simulink model "Mmc"  (R2024b)
settings: Solver=ode23t  StartTime=0.0  StopTime=2  FixedStep=Ts_Power
values from neighbouring files (symbols this model uses):
  Ch = 0.94e-6*ones(4,3)    [MmcParameters.m]
  Cm = 0.55e-3    (= 0.00055)    [MmcParameters.m]
  Cmo = 0.55e-3*ones(4,3)    [MmcParameters.m]
  eta = N*delta_wmax*Vmax^2/(P_rated*sin(phi_r)-Q_rated*cos(phi_r))    [MmcParameters.m]
  Fnom = 50    [MmcParameters.m]
  fs = 20000    [MmcParameters.m]
  I_b = Snom/Vnom_AC/sqrt(3)    [MmcParameters.m]
  Ipp_b = Snom/Vnom_AC/sqrt(3/2)    [MmcParameters.m]
  kicir = R0*alpha_ic    (= 62831.8530718)    [MmcParameters.m]
  kpcir = L0*alpha_ic    (= 1012.64003201)    [MmcParameters.m]
  L0 = (4.67e-3+5e-3)    (= 0.00967)    [MmcParameters.m]
  mu = eta*4/((2*Vmax^2-V0^2)^2-V0^4)*(P_rated*cos(phi_r)+Q_rated*sin(phi_r))/N    [MmcParameters.m]
  Nb_PM = 2    [MmcParameters.m]
  phi_r = pi/2    (= 1.57079632679)    [MmcParameters.m]
  R0 = 0.1+0.5    (= 0.6)    [MmcParameters.m]
  Rdis = 1e6*ones(4,3)    [MmcParameters.m]
  Rh = 1e-3./(2*pi*1000*Ch)    [MmcParameters.m]
  Rm = 0.2./(2*pi*120*Cmo)    [MmcParameters.m]
  SCR = 10    [MmcParameters.m]
  SigmaM = 10    [MmcParameters.m]
  Snom = 20*Vnom_AC*sqrt(3)    [MmcParameters.m]
  Ts_Power = 5e-7    (= 5e-07)    [MmcParameters.m]
  V0 = 1    [MmcParameters.m]
  V_b = Vnom_AC    (= 400)    [MmcParameters.m]
  VDCm = 480/2    (= 240)    [MmcParameters.m]
  VDCp = 480/2    (= 240)    [MmcParameters.m]
  Vnom_AC = 400    [MmcParameters.m]
  Vnom_PM = 480/2    (= 240)    [MmcParameters.m]
  w_b = 2*pi*Fnom    (= 314.159265359)    [MmcParameters.m]
  Zn = Vnom_AC^2 / Snom    [MmcParameters.m]
undefined symbols (not defined in the file or in its folder): DiscIntNeverNeededParam
libraries: spsIGBTDiodeLib x48, spsSeriesRLCBranchLib x42, spsVoltageMeasurementLib x16, spsTriangleGeneratorLib x12, spsCurrentMeasurementLib x7, spsFirstOrderFilterLib x6, eePwmGeneratorMultilevel x6, spsabctodq0Lib x3, spsGroundLib x2, spsMeanLib x2, spsDCVoltageSourceLib x2, spsThreePhaseVIMeasurementLib x2
(part 2 of 3)

== system Mmc/MMC/Full-bridge/HBua2 ==
  gates : Inport
  Ch : spsSeriesRLCBranchLib/Series RLC Branch  LConnTagsString=__new0  RConnTagsString=__new0  BranchType=RC  Resistance=Rh(2,1)  Inductance=1e-3  SetiL0=off  InitialCurrent=0  Capacitance=Ch(2,1)  Setx0=off  InitialVoltage=750  Measurements=None
  Cm : spsSeriesRLCBranchLib/Series RLC Branch  LConnTagsString=__new0  RConnTagsString=__new0  BranchType=RC  Resistance=Rm(2,1)  Inductance=1e-3  SetiL0=off  InitialCurrent=0  Capacitance=Cmo(2,1)  Setx0=on  InitialVoltage=20  Measurements=None
  Demux1 : Demux
  IGBT/Diode{,1..3} (4 alike) : spsIGBTDiodeLib/IGBT//Diode  Ron=Ron  Rs=Rs  Cs=Cs  Measurements=off
  Rdis : spsSeriesRLCBranchLib/Series RLC Branch  LConnTagsString=__new0  RConnTagsString=__new0  BranchType=R  Resistance=Rdis(2,1)  Inductance=1e-3  SetiL0=off  InitialCurrent=0  Capacitance=Cm  Setx0=off  InitialVoltage=750  Measurements=None
  VA : PMIOPort  Side=Left
  VB : PMIOPort  Port=2  Side=Left
  DC+ : PMIOPort  Port=3  Side=Right
  DC- : PMIOPort  Port=4  Side=Right
  wires:
  gates/1 -> Demux1/1
  Demux1/4 -> IGBT/Diode3/1
  Demux1/3 -> IGBT/Diode2/1
  Demux1/2 -> IGBT/Diode1/1
  Demux1/1 -> IGBT/Diode/1
  connections:
  IGBT/Diode3/LConn1 -- VB/RConn1 -- IGBT/Diode2/RConn1
  Ch/LConn1 -- Rdis/LConn1 -- DC+/RConn1 -- IGBT/Diode/LConn1 -- IGBT/Diode2/LConn1 -- Cm/LConn1
  IGBT/Diode/RConn1 -- VA/RConn1 -- IGBT/Diode1/LConn1
  Ch/RConn1 -- DC-/RConn1 -- Rdis/RConn1 -- Cm/RConn1 -- IGBT/Diode3/RConn1 -- IGBT/Diode1/RConn1

== system Mmc/MMC/Full-bridge 1/HBua1 ==
  gates : Inport
  Ch : spsSeriesRLCBranchLib/Series RLC Branch  LConnTagsString=__new0  RConnTagsString=__new0  BranchType=RC  Resistance=Rh(2,1)  Inductance=1e-3  SetiL0=off  InitialCurrent=0  Capacitance=Ch(2,1)  Setx0=off  InitialVoltage=750  Measurements=None
  Cm : spsSeriesRLCBranchLib/Series RLC Branch  LConnTagsString=__new0  RConnTagsString=__new0  BranchType=RC  Resistance=Rm(2,1)  Inductance=1e-3  SetiL0=off  InitialCurrent=0  Capacitance=Cmo(2,1)  Setx0=on  InitialVoltage=20  Measurements=None
  Demux1 : Demux
  IGBT/Diode{,1..3} (4 alike) : spsIGBTDiodeLib/IGBT//Diode  Ron=Ron  Rs=Rs  Cs=Cs  Measurements=off
  Rdis : spsSeriesRLCBranchLib/Series RLC Branch  LConnTagsString=__new0  RConnTagsString=__new0  BranchType=R  Resistance=Rdis(2,1)  Inductance=1e-3  SetiL0=off  InitialCurrent=0  Capacitance=Cm  Setx0=off  InitialVoltage=750  Measurements=None
  VA : PMIOPort  Side=Left
  VB : PMIOPort  Port=2  Side=Left
  DC+ : PMIOPort  Port=3  Side=Right
  DC- : PMIOPort  Port=4  Side=Right
  wires:
  gates/1 -> Demux1/1
  Demux1/4 -> IGBT/Diode3/1
  Demux1/3 -> IGBT/Diode2/1
  Demux1/2 -> IGBT/Diode1/1
  Demux1/1 -> IGBT/Diode/1
  connections:
  IGBT/Diode3/LConn1 -- VB/RConn1 -- IGBT/Diode2/RConn1
  Ch/LConn1 -- Rdis/LConn1 -- DC+/RConn1 -- IGBT/Diode/LConn1 -- IGBT/Diode2/LConn1 -- Cm/LConn1
  IGBT/Diode/RConn1 -- VA/RConn1 -- IGBT/Diode1/LConn1
  Ch/RConn1 -- DC-/RConn1 -- Rdis/RConn1 -- Cm/RConn1 -- IGBT/Diode3/RConn1 -- IGBT/Diode1/RConn1

== system Mmc/MMC/Full-bridge 1/HBua2 ==
  gates : Inport
  Ch : spsSeriesRLCBranchLib/Series RLC Branch  LConnTagsString=__new0  RConnTagsString=__new0  BranchType=RC  Resistance=Rh(2,1)  Inductance=1e-3  SetiL0=off  InitialCurrent=0  Capacitance=Ch(2,1)  Setx0=off  InitialVoltage=750  Measurements=None
  Cm : spsSeriesRLCBranchLib/Series RLC Branch  LConnTagsString=__new0  RConnTagsString=__new0  BranchType=RC  Resistance=Rm(2,1)  Inductance=1e-3  SetiL0=off  InitialCurrent=0  Capacitance=Cmo(2,1)  Setx0=on  InitialVoltage=20  Measurements=None
  Demux1 : Demux
  IGBT/Diode{,1..3} (4 alike) : spsIGBTDiodeLib/IGBT//Diode  Ron=Ron  Rs=Rs  Cs=Cs  Measurements=off
  Rdis : spsSeriesRLCBranchLib/Series RLC Branch  LConnTagsString=__new0  RConnTagsString=__new0  BranchType=R  Resistance=Rdis(2,1)  Inductance=1e-3  SetiL0=off  InitialCurrent=0  Capacitance=Cm  Setx0=off  InitialVoltage=750  Measurements=None
  VA : PMIOPort  Side=Left
  VB : PMIOPort  Port=2  Side=Left
  DC+ : PMIOPort  Port=3  Side=Right
  DC- : PMIOPort  Port=4  Side=Right
  wires:
  gates/1 -> Demux1/1
  Demux1/4 -> IGBT/Diode3/1
  Demux1/3 -> IGBT/Diode2/1
  Demux1/2 -> IGBT/Diode1/1
  Demux1/1 -> IGBT/Diode/1
  connections:
  IGBT/Diode3/LConn1 -- VB/RConn1 -- IGBT/Diode2/RConn1
  Ch/LConn1 -- Rdis/LConn1 -- DC+/RConn1 -- IGBT/Diode/LConn1 -- IGBT/Diode2/LConn1 -- Cm/LConn1
  IGBT/Diode/RConn1 -- VA/RConn1 -- IGBT/Diode1/LConn1
  Ch/RConn1 -- DC-/RConn1 -- Rdis/RConn1 -- Cm/RConn1 -- IGBT/Diode3/RConn1 -- IGBT/Diode1/RConn1

== system Mmc/MMC/Full-bridge 2/HBua1 ==
  gates : Inport
  Ch : spsSeriesRLCBranchLib/Series RLC Branch  LConnTagsString=__new0  RConnTagsString=__new0  BranchType=RC  Resistance=Rh(2,1)  Inductance=1e-3  SetiL0=off  InitialCurrent=0  Capacitance=Ch(2,1)  Setx0=off  InitialVoltage=750  Measurements=None
  Cm : spsSeriesRLCBranchLib/Series RLC Branch  LConnTagsString=__new0  RConnTagsString=__new0  BranchType=RC  Resistance=Rm(2,1)  Inductance=1e-3  SetiL0=off  InitialCurrent=0  Capacitance=Cmo(2,1)  Setx0=on  InitialVoltage=20  Measurements=None
  Demux1 : Demux
  IGBT/Diode{,1..3} (4 alike) : spsIGBTDiodeLib/IGBT//Diode  Ron=Ron  Rs=Rs  Cs=Cs  Measurements=off
  Rdis : spsSeriesRLCBranchLib/Series RLC Branch  LConnTagsString=__new0  RConnTagsString=__new0  BranchType=R  Resistance=Rdis(2,1)  Inductance=1e-3  SetiL0=off  InitialCurrent=0  Capacitance=Cm  Setx0=off  InitialVoltage=750  Measurements=None
  VA : PMIOPort  Side=Left
  VB : PMIOPort  Port=2  Side=Left
  DC+ : PMIOPort  Port=3  Side=Right
  DC- : PMIOPort  Port=4  Side=Right
  wires:
  gates/1 -> Demux1/1
  Demux1/4 -> IGBT/Diode3/1
  Demux1/3 -> IGBT/Diode2/1
  Demux1/2 -> IGBT/Diode1/1
  Demux1/1 -> IGBT/Diode/1
  connections:
  IGBT/Diode3/LConn1 -- VB/RConn1 -- IGBT/Diode2/RConn1
  Ch/LConn1 -- Rdis/LConn1 -- DC+/RConn1 -- IGBT/Diode/LConn1 -- IGBT/Diode2/LConn1 -- Cm/LConn1
  IGBT/Diode/RConn1 -- VA/RConn1 -- IGBT/Diode1/LConn1
  Ch/RConn1 -- DC-/RConn1 -- Rdis/RConn1 -- Cm/RConn1 -- IGBT/Diode3/RConn1 -- IGBT/Diode1/RConn1

== system Mmc/MMC/Full-bridge 2/HBua2 ==
  gates : Inport
  Ch : spsSeriesRLCBranchLib/Series RLC Branch  LConnTagsString=__new0  RConnTagsString=__new0  BranchType=RC  Resistance=Rh(2,1)  Inductance=1e-3  SetiL0=off  InitialCurrent=0  Capacitance=Ch(2,1)  Setx0=off  InitialVoltage=750  Measurements=None
  Cm : spsSeriesRLCBranchLib/Series RLC Branch  LConnTagsString=__new0  RConnTagsString=__new0  BranchType=RC  Resistance=Rm(2,1)  Inductance=1e-3  SetiL0=off  InitialCurrent=0  Capacitance=Cmo(2,1)  Setx0=on  InitialVoltage=20  Measurements=None
  Demux1 : Demux
  IGBT/Diode{,1..3} (4 alike) : spsIGBTDiodeLib/IGBT//Diode  Ron=Ron  Rs=Rs  Cs=Cs  Measurements=off
  Rdis : spsSeriesRLCBranchLib/Series RLC Branch  LConnTagsString=__new0  RConnTagsString=__new0  BranchType=R  Resistance=Rdis(2,1)  Inductance=1e-3  SetiL0=off  InitialCurrent=0  Capacitance=Cm  Setx0=off  InitialVoltage=750  Measurements=None
  VA : PMIOPort  Side=Left
  VB : PMIOPort  Port=2  Side=Left
  DC+ : PMIOPort  Port=3  Side=Right
  DC- : PMIOPort  Port=4  Side=Right
  wires:
  gates/1 -> Demux1/1
  Demux1/4 -> IGBT/Diode3/1
  Demux1/3 -> IGBT/Diode2/1
  Demux1/2 -> IGBT/Diode1/1
  Demux1/1 -> IGBT/Diode/1
  connections:
  IGBT/Diode3/LConn1 -- VB/RConn1 -- IGBT/Diode2/RConn1
  Ch/LConn1 -- Rdis/LConn1 -- DC+/RConn1 -- IGBT/Diode/LConn1 -- IGBT/Diode2/LConn1 -- Cm/LConn1
  IGBT/Diode/RConn1 -- VA/RConn1 -- IGBT/Diode1/LConn1
  Ch/RConn1 -- DC-/RConn1 -- Rdis/RConn1 -- Cm/RConn1 -- IGBT/Diode3/RConn1 -- IGBT/Diode1/RConn1

== system Mmc/MMC/Full-bridge 3/HBua1 ==
  gates : Inport
  Ch : spsSeriesRLCBranchLib/Series RLC Branch  LConnTagsString=__new0  RConnTagsString=__new0  BranchType=RC  Resistance=Rh(2,1)  Inductance=1e-3  SetiL0=off  InitialCurrent=0  Capacitance=Ch(2,1)  Setx0=off  InitialVoltage=750  Measurements=None
  Cm : spsSeriesRLCBranchLib/Series RLC Branch  LConnTagsString=__new0  RConnTagsString=__new0  BranchType=RC  Resistance=Rm(2,1)  Inductance=1e-3  SetiL0=off  InitialCurrent=0  Capacitance=Cmo(2,1)  Setx0=on  InitialVoltage=20  Measurements=None
  Demux1 : Demux
  IGBT/Diode{,1..3} (4 alike) : spsIGBTDiodeLib/IGBT//Diode  Ron=Ron  Rs=Rs  Cs=Cs  Measurements=off
  Rdis : spsSeriesRLCBranchLib/Series RLC Branch  LConnTagsString=__new0  RConnTagsString=__new0  BranchType=R  Resistance=Rdis(2,1)  Inductance=1e-3  SetiL0=off  InitialCurrent=0  Capacitance=Cm  Setx0=off  InitialVoltage=750  Measurements=None
  VA : PMIOPort  Side=Left
  VB : PMIOPort  Port=2  Side=Left
  DC+ : PMIOPort  Port=3  Side=Right
  DC- : PMIOPort  Port=4  Side=Right
  wires:
  gates/1 -> Demux1/1
  Demux1/4 -> IGBT/Diode3/1
  Demux1/3 -> IGBT/Diode2/1
  Demux1/2 -> IGBT/Diode1/1
  Demux1/1 -> IGBT/Diode/1
  connections:
  IGBT/Diode3/LConn1 -- VB/RConn1 -- IGBT/Diode2/RConn1
  Ch/LConn1 -- Rdis/LConn1 -- DC+/RConn1 -- IGBT/Diode/LConn1 -- IGBT/Diode2/LConn1 -- Cm/LConn1
  IGBT/Diode/RConn1 -- VA/RConn1 -- IGBT/Diode1/LConn1
  Ch/RConn1 -- DC-/RConn1 -- Rdis/RConn1 -- Cm/RConn1 -- IGBT/Diode3/RConn1 -- IGBT/Diode1/RConn1

== system Mmc/MMC/Full-bridge 3/HBua2 ==
  gates : Inport
  Ch : spsSeriesRLCBranchLib/Series RLC Branch  LConnTagsString=__new0  RConnTagsString=__new0  BranchType=RC  Resistance=Rh(2,1)  Inductance=1e-3  SetiL0=off  InitialCurrent=0  Capacitance=Ch(2,1)  Setx0=off  InitialVoltage=750  Measurements=None
  Cm : spsSeriesRLCBranchLib/Series RLC Branch  LConnTagsString=__new0  RConnTagsString=__new0  BranchType=RC  Resistance=Rm(2,1)  Inductance=1e-3  SetiL0=off  InitialCurrent=0  Capacitance=Cmo(2,1)  Setx0=on  InitialVoltage=20  Measurements=None
  Demux1 : Demux
  IGBT/Diode{,1..3} (4 alike) : spsIGBTDiodeLib/IGBT//Diode  Ron=Ron  Rs=Rs  Cs=Cs  Measurements=off
  Rdis : spsSeriesRLCBranchLib/Series RLC Branch  LConnTagsString=__new0  RConnTagsString=__new0  BranchType=R  Resistance=Rdis(2,1)  Inductance=1e-3  SetiL0=off  InitialCurrent=0  Capacitance=Cm  Setx0=off  InitialVoltage=750  Measurements=None
  VA : PMIOPort  Side=Left
  VB : PMIOPort  Port=2  Side=Left
  DC+ : PMIOPort  Port=3  Side=Right
  DC- : PMIOPort  Port=4  Side=Right
  wires:
  gates/1 -> Demux1/1
  Demux1/4 -> IGBT/Diode3/1
  Demux1/3 -> IGBT/Diode2/1
  Demux1/2 -> IGBT/Diode1/1
  Demux1/1 -> IGBT/Diode/1
  connections:
  IGBT/Diode3/LConn1 -- VB/RConn1 -- IGBT/Diode2/RConn1
  Ch/LConn1 -- Rdis/LConn1 -- DC+/RConn1 -- IGBT/Diode/LConn1 -- IGBT/Diode2/LConn1 -- Cm/LConn1
  IGBT/Diode/RConn1 -- VA/RConn1 -- IGBT/Diode1/LConn1
  Ch/RConn1 -- DC-/RConn1 -- Rdis/RConn1 -- Cm/RConn1 -- IGBT/Diode3/RConn1 -- IGBT/Diode1/RConn1

== system Mmc/MMC/Full-bridge 4/HBua1 ==
  gates : Inport
  Ch : spsSeriesRLCBranchLib/Series RLC Branch  LConnTagsString=__new0  RConnTagsString=__new0  BranchType=RC  Resistance=Rh(2,1)  Inductance=1e-3  SetiL0=off  InitialCurrent=0  Capacitance=Ch(2,1)  Setx0=off  InitialVoltage=750  Measurements=None
  Cm : spsSeriesRLCBranchLib/Series RLC Branch  LConnTagsString=__new0  RConnTagsString=__new0  BranchType=RC  Resistance=Rm(2,1)  Inductance=1e-3  SetiL0=off  InitialCurrent=0  Capacitance=Cmo(2,1)  Setx0=on  InitialVoltage=20  Measurements=None
  Demux1 : Demux
  IGBT/Diode{,1..3} (4 alike) : spsIGBTDiodeLib/IGBT//Diode  Ron=Ron  Rs=Rs  Cs=Cs  Measurements=off
  Rdis : spsSeriesRLCBranchLib/Series RLC Branch  LConnTagsString=__new0  RConnTagsString=__new0  BranchType=R  Resistance=Rdis(2,1)  Inductance=1e-3  SetiL0=off  InitialCurrent=0  Capacitance=Cm  Setx0=off  InitialVoltage=750  Measurements=None
  VA : PMIOPort  Side=Left
  VB : PMIOPort  Port=2  Side=Left
  DC+ : PMIOPort  Port=3  Side=Right
  DC- : PMIOPort  Port=4  Side=Right
  wires:
  gates/1 -> Demux1/1
  Demux1/4 -> IGBT/Diode3/1
  Demux1/3 -> IGBT/Diode2/1
  Demux1/2 -> IGBT/Diode1/1
  Demux1/1 -> IGBT/Diode/1
  connections:
  IGBT/Diode3/LConn1 -- VB/RConn1 -- IGBT/Diode2/RConn1
  Ch/LConn1 -- Rdis/LConn1 -- DC+/RConn1 -- IGBT/Diode/LConn1 -- IGBT/Diode2/LConn1 -- Cm/LConn1
  IGBT/Diode/RConn1 -- VA/RConn1 -- IGBT/Diode1/LConn1
  Ch/RConn1 -- DC-/RConn1 -- Rdis/RConn1 -- Cm/RConn1 -- IGBT/Diode3/RConn1 -- IGBT/Diode1/RConn1

== system Mmc/MMC/Full-bridge 4/HBua2 ==
  gates : Inport
  Ch : spsSeriesRLCBranchLib/Series RLC Branch  LConnTagsString=__new0  RConnTagsString=__new0  BranchType=RC  Resistance=Rh(2,1)  Inductance=1e-3  SetiL0=off  InitialCurrent=0  Capacitance=Ch(2,1)  Setx0=off  InitialVoltage=750  Measurements=None
  Cm : spsSeriesRLCBranchLib/Series RLC Branch  LConnTagsString=__new0  RConnTagsString=__new0  BranchType=RC  Resistance=Rm(2,1)  Inductance=1e-3  SetiL0=off  InitialCurrent=0  Capacitance=Cmo(2,1)  Setx0=on  InitialVoltage=20  Measurements=None
  Demux1 : Demux
  IGBT/Diode{,1..3} (4 alike) : spsIGBTDiodeLib/IGBT//Diode  Ron=Ron  Rs=Rs  Cs=Cs  Measurements=off
  Rdis : spsSeriesRLCBranchLib/Series RLC Branch  LConnTagsString=__new0  RConnTagsString=__new0  BranchType=R  Resistance=Rdis(2,1)  Inductance=1e-3  SetiL0=off  InitialCurrent=0  Capacitance=Cm  Setx0=off  InitialVoltage=750  Measurements=None
  VA : PMIOPort  Side=Left
  VB : PMIOPort  Port=2  Side=Left
  DC+ : PMIOPort  Port=3  Side=Right
  DC- : PMIOPort  Port=4  Side=Right
  wires:
  gates/1 -> Demux1/1
  Demux1/4 -> IGBT/Diode3/1
  Demux1/3 -> IGBT/Diode2/1
  Demux1/2 -> IGBT/Diode1/1
  Demux1/1 -> IGBT/Diode/1
  connections:
  IGBT/Diode3/LConn1 -- VB/RConn1 -- IGBT/Diode2/RConn1
  Ch/LConn1 -- Rdis/LConn1 -- DC+/RConn1 -- IGBT/Diode/LConn1 -- IGBT/Diode2/LConn1 -- Cm/LConn1
  IGBT/Diode/RConn1 -- VA/RConn1 -- IGBT/Diode1/LConn1
  Ch/RConn1 -- DC-/RConn1 -- Rdis/RConn1 -- Cm/RConn1 -- IGBT/Diode3/RConn1 -- IGBT/Diode1/RConn1

== system Mmc/MMC/Full-bridge 5/HBua1 ==
  gates : Inport
  Ch : spsSeriesRLCBranchLib/Series RLC Branch  LConnTagsString=__new0  RConnTagsString=__new0  BranchType=RC  Resistance=Rh(2,1)  Inductance=1e-3  SetiL0=off  InitialCurrent=0  Capacitance=Ch(2,1)  Setx0=off  InitialVoltage=750  Measurements=None
  Cm : spsSeriesRLCBranchLib/Series RLC Branch  LConnTagsString=__new0  RConnTagsString=__new0  BranchType=RC  Resistance=Rm(2,1)  Inductance=1e-3  SetiL0=off  InitialCurrent=0  Capacitance=Cmo(2,1)  Setx0=on  InitialVoltage=20  Measurements=None
  Demux1 : Demux
  IGBT/Diode{,1..3} (4 alike) : spsIGBTDiodeLib/IGBT//Diode  Ron=Ron  Rs=Rs  Cs=Cs  Measurements=off
  Rdis : spsSeriesRLCBranchLib/Series RLC Branch  LConnTagsString=__new0  RConnTagsString=__new0  BranchType=R  Resistance=Rdis(2,1)  Inductance=1e-3  SetiL0=off  InitialCurrent=0  Capacitance=Cm  Setx0=off  InitialVoltage=750  Measurements=None
  VA : PMIOPort  Side=Left
  VB : PMIOPort  Port=2  Side=Left
  DC+ : PMIOPort  Port=3  Side=Right
  DC- : PMIOPort  Port=4  Side=Right
  wires:
  gates/1 -> Demux1/1
  Demux1/4 -> IGBT/Diode3/1
  Demux1/3 -> IGBT/Diode2/1
  Demux1/2 -> IGBT/Diode1/1
  Demux1/1 -> IGBT/Diode/1
  connections:
  IGBT/Diode3/LConn1 -- VB/RConn1 -- IGBT/Diode2/RConn1
  Ch/LConn1 -- Rdis/LConn1 -- DC+/RConn1 -- IGBT/Diode/LConn1 -- IGBT/Diode2/LConn1 -- Cm/LConn1
  IGBT/Diode/RConn1 -- VA/RConn1 -- IGBT/Diode1/LConn1
  Ch/RConn1 -- DC-/RConn1 -- Rdis/RConn1 -- Cm/RConn1 -- IGBT/Diode3/RConn1 -- IGBT/Diode1/RConn1

== system Mmc/MMC/Full-bridge 5/HBua2 ==
  gates : Inport
  Ch : spsSeriesRLCBranchLib/Series RLC Branch  LConnTagsString=__new0  RConnTagsString=__new0  BranchType=RC  Resistance=Rh(2,1)  Inductance=1e-3  SetiL0=off  InitialCurrent=0  Capacitance=Ch(2,1)  Setx0=off  InitialVoltage=750  Measurements=None
  Cm : spsSeriesRLCBranchLib/Series RLC Branch  LConnTagsString=__new0  RConnTagsString=__new0  BranchType=RC  Resistance=Rm(2,1)  Inductance=1e-3  SetiL0=off  InitialCurrent=0  Capacitance=Cmo(2,1)  Setx0=on  InitialVoltage=20  Measurements=None
  Demux1 : Demux
  IGBT/Diode{,1..3} (4 alike) : spsIGBTDiodeLib/IGBT//Diode  Ron=Ron  Rs=Rs  Cs=Cs  Measurements=off
  Rdis : spsSeriesRLCBranchLib/Series RLC Branch  LConnTagsString=__new0  RConnTagsString=__new0  BranchType=R  Resistance=Rdis(2,1)  Inductance=1e-3  SetiL0=off  InitialCurrent=0  Capacitance=Cm  Setx0=off  InitialVoltage=750  Measurements=None
  VA : PMIOPort  Side=Left
  VB : PMIOPort  Port=2  Side=Left
  DC+ : PMIOPort  Port=3  Side=Right
  DC- : PMIOPort  Port=4  Side=Right
  wires:
  gates/1 -> Demux1/1
  Demux1/4 -> IGBT/Diode3/1
  Demux1/3 -> IGBT/Diode2/1
  Demux1/2 -> IGBT/Diode1/1
  Demux1/1 -> IGBT/Diode/1
  connections:
  IGBT/Diode3/LConn1 -- VB/RConn1 -- IGBT/Diode2/RConn1
  Ch/LConn1 -- Rdis/LConn1 -- DC+/RConn1 -- IGBT/Diode/LConn1 -- IGBT/Diode2/LConn1 -- Cm/LConn1
  IGBT/Diode/RConn1 -- VA/RConn1 -- IGBT/Diode1/LConn1
  Ch/RConn1 -- DC-/RConn1 -- Rdis/RConn1 -- Cm/RConn1 -- IGBT/Diode3/RConn1 -- IGBT/Diode1/RConn1

== system Mmc/MMC/PS-PWM/PS-PWM lower a ==
  ref : Inport
  Gain : Gain  Gain=70
  Gain1 : Gain  Gain=70
  Logical Operator : Logic  Operator=NOT  AllPortsSameDT=off  OutDataTypeStr=boolean
  Logical Operator1 : Logic  Operator=NOT  AllPortsSameDT=off  OutDataTypeStr=boolean
  Mux : Mux
  Relational Operator : RelationalOperator  OutDataTypeStr=boolean  RndMeth=Simplest  InputSameDT=off
  Relational Operator1 : RelationalOperator  OutDataTypeStr=boolean  RndMeth=Simplest  InputSameDT=off
  Triangle Generator : spsTriangleGeneratorLib/Triangle Generator  Freq=1e3  Phase=0  Ts=Ts_Power
  Triangle Generator1 : spsTriangleGeneratorLib/Triangle Generator  Freq=1e3  Phase=pi/(4)  Ts=Ts_Power
  Ppa : Outport
  wires:
  Logical Operator/1 -> Mux/2
  ref/1 -> Relational Operator1/1, Relational Operator/1
  Relational Operator/1 -> Mux/1, Logical Operator/1
  Relational Operator1/1 -> Logical Operator1/1, Mux/3
  Triangle Generator/1 -> Gain/1
  Triangle Generator1/1 -> Gain1/1
  Mux/1 -> Ppa/1
  Logical Operator1/1 -> Mux/4
  Gain1/1 -> Relational Operator1/2
  Gain/1 -> Relational Operator/2

== system Mmc/MMC/PS-PWM/PS-PWM lower b ==
  ref : Inport
  Gain : Gain  Gain=70
  Gain1 : Gain  Gain=70
  Logical Operator : Logic  Operator=NOT  AllPortsSameDT=off  OutDataTypeStr=boolean
  Logical Operator1 : Logic  Operator=NOT  AllPortsSameDT=off  OutDataTypeStr=boolean
  Mux : Mux
  Relational Operator : RelationalOperator  OutDataTypeStr=boolean  RndMeth=Simplest  InputSameDT=off
  Relational Operator1 : RelationalOperator  OutDataTypeStr=boolean  RndMeth=Simplest  InputSameDT=off
  Triangle Generator : spsTriangleGeneratorLib/Triangle Generator  Freq=1e3  Phase=0  Ts=Ts_Power
  Triangle Generator1 : spsTriangleGeneratorLib/Triangle Generator  Freq=1e3  Phase=pi/(4)  Ts=Ts_Power
  Ppa : Outport
  wires:
  Logical Operator/1 -> Mux/2
  ref/1 -> Relational Operator1/1, Relational Operator/1
  Relational Operator/1 -> Mux/1, Logical Operator/1
  Relational Operator1/1 -> Logical Operator1/1, Mux/3
  Triangle Generator/1 -> Gain/1
  Triangle Generator1/1 -> Gain1/1
  Mux/1 -> Ppa/1
  Logical Operator1/1 -> Mux/4
  Gain/1 -> Relational Operator/2
  Gain1/1 -> Relational Operator1/2

== system Mmc/MMC/PS-PWM/PS-PWM lower c ==
  ref : Inport
  Gain : Gain  Gain=70
  Gain1 : Gain  Gain=70
  Logical Operator : Logic  Operator=NOT  AllPortsSameDT=off  OutDataTypeStr=boolean
  Logical Operator1 : Logic  Operator=NOT  AllPortsSameDT=off  OutDataTypeStr=boolean
  Mux : Mux
  Relational Operator : RelationalOperator  OutDataTypeStr=boolean  RndMeth=Simplest  InputSameDT=off
  Relational Operator1 : RelationalOperator  OutDataTypeStr=boolean  RndMeth=Simplest  InputSameDT=off
  Triangle Generator : spsTriangleGeneratorLib/Triangle Generator  Freq=1e3  Phase=0  Ts=Ts_Power
  Triangle Generator1 : spsTriangleGeneratorLib/Triangle Generator  Freq=1e3  Phase=pi/(4)  Ts=Ts_Power
  Ppa : Outport
  wires:
  Logical Operator/1 -> Mux/2
  ref/1 -> Relational Operator1/1, Relational Operator/1
  Relational Operator/1 -> Mux/1, Logical Operator/1
  Relational Operator1/1 -> Logical Operator1/1, Mux/3
  Triangle Generator/1 -> Gain/1
  Triangle Generator1/1 -> Gain1/1
  Mux/1 -> Ppa/1
  Logical Operator1/1 -> Mux/4
  Gain/1 -> Relational Operator/2
  Gain1/1 -> Relational Operator1/2

== system Mmc/MMC/PS-PWM/PS-PWM upper a ==
  ref : Inport
  Gain : Gain  Gain=70
  Gain1 : Gain  Gain=70
  Logical Operator : Logic  Operator=NOT  AllPortsSameDT=off  OutDataTypeStr=boolean
  Logical Operator1 : Logic  Operator=NOT  AllPortsSameDT=off  OutDataTypeStr=boolean
  Mux : Mux
  Relational Operator : RelationalOperator  OutDataTypeStr=boolean  RndMeth=Simplest  InputSameDT=off
  Relational Operator1 : RelationalOperator  OutDataTypeStr=boolean  RndMeth=Simplest  InputSameDT=off
  Scope : Scope
  Triangle Generator : spsTriangleGeneratorLib/Triangle Generator  Freq=1e3  Phase=0  Ts=Ts_Power
  Triangle Generator1 : spsTriangleGeneratorLib/Triangle Generator  Freq=1e3  Phase=pi/(4)  Ts=Ts_Power
  Ppa : Outport
  wires:
  Triangle Generator1/1 -> Gain1/1
  Triangle Generator/1 -> Gain/1
  ref/1 -> Scope/1, Relational Operator1/1, Relational Operator/1
  Mux/1 -> Ppa/1
  Relational Operator/1 -> Mux/1, Logical Operator/1
  Relational Operator1/1 -> Logical Operator1/1, Mux/3
  Logical Operator/1 -> Mux/2
  Logical Operator1/1 -> Mux/4
  Gain/1 -> Relational Operator/2
  Gain1/1 -> Relational Operator1/2

== system Mmc/MMC/PS-PWM/PS-PWM upper b ==
  ref : Inport
  Gain : Gain  Gain=70
  Gain1 : Gain  Gain=70
  Logical Operator : Logic  Operator=NOT  AllPortsSameDT=off  OutDataTypeStr=boolean
  Logical Operator1 : Logic  Operator=NOT  AllPortsSameDT=off  OutDataTypeStr=boolean
  Mux : Mux
  Relational Operator : RelationalOperator  OutDataTypeStr=boolean  RndMeth=Simplest  InputSameDT=off
  Relational Operator1 : RelationalOperator  OutDataTypeStr=boolean  RndMeth=Simplest  InputSameDT=off
  Triangle Generator : spsTriangleGeneratorLib/Triangle Generator  Freq=1e3  Phase=0  Ts=Ts_Power
  Triangle Generator1 : spsTriangleGeneratorLib/Triangle Generator  Freq=1e3  Phase=pi/(4)  Ts=Ts_Power
  Ppa : Outport
  wires:
  Triangle Generator1/1 -> Gain1/1
  Triangle Generator/1 -> Gain/1
  ref/1 -> Relational Operator1/1, Relational Operator/1
  Mux/1 -> Ppa/1
  Relational Operator/1 -> Mux/1, Logical Operator/1
  Relational Operator1/1 -> Logical Operator1/1, Mux/3
  Logical Operator/1 -> Mux/2
  Logical Operator1/1 -> Mux/4
  Gain/1 -> Relational Operator/2
  Gain1/1 -> Relational Operator1/2

== system Mmc/MMC/PS-PWM/PS-PWM upper c ==
  ref : Inport
  Gain : Gain  Gain=70
  Gain1 : Gain  Gain=70
  Logical Operator : Logic  Operator=NOT  AllPortsSameDT=off  OutDataTypeStr=boolean
  Logical Operator1 : Logic  Operator=NOT  AllPortsSameDT=off  OutDataTypeStr=boolean
  Mux : Mux
  Relational Operator : RelationalOperator  OutDataTypeStr=boolean  RndMeth=Simplest  InputSameDT=off
  Relational Operator1 : RelationalOperator  OutDataTypeStr=boolean  RndMeth=Simplest  InputSameDT=off
  Triangle Generator : spsTriangleGeneratorLib/Triangle Generator  Freq=1e3  Phase=0  Ts=Ts_Power
  Triangle Generator1 : spsTriangleGeneratorLib/Triangle Generator  Freq=1e3  Phase=pi/(4)  Ts=Ts_Power
  Ppa : Outport
  wires:
  Triangle Generator1/1 -> Gain1/1
  Triangle Generator/1 -> Gain/1
  ref/1 -> Relational Operator1/1, Relational Operator/1
  Mux/1 -> Ppa/1
  Relational Operator/1 -> Mux/1, Logical Operator/1
  Relational Operator1/1 -> Logical Operator1/1, Mux/3
  Logical Operator/1 -> Mux/2
  Logical Operator1/1 -> Mux/4
  Gain/1 -> Relational Operator/2
  Gain1/1 -> Relational Operator1/2

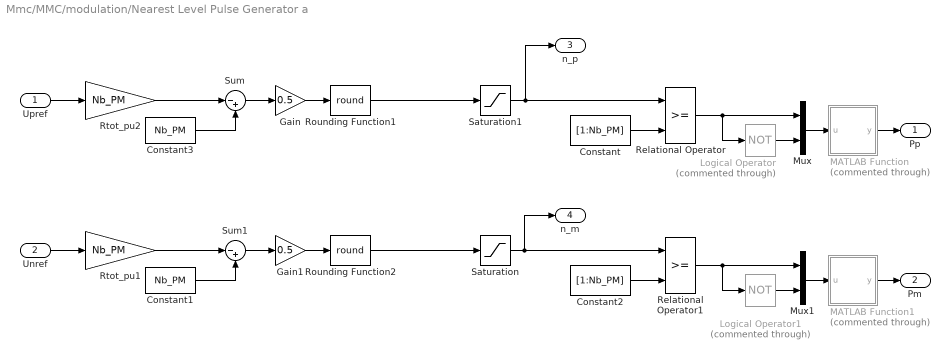
== system Mmc/MMC/modulation/Nearest Level Pulse Generator a  ==
  Upref : Inport
  Unref : Inport  Port=2
  Constant : Constant  Value=[1:Nb_PM]
  Constant1 : Constant  Value=Nb_PM
  Constant2 : Constant  Value=[1:Nb_PM]
  Constant3 : Constant  Value=Nb_PM
  Gain : Gain  Gain=0.5
  Gain1 : Gain  Gain=0.5
  Logical Operator : Logic  Commented=through  Operator=NOT  AllPortsSameDT=off  OutDataTypeStr=float('double')
  Logical Operator1 : Logic  Commented=through  Operator=NOT  AllPortsSameDT=off  OutDataTypeStr=float('double')
  MATLAB Function : MATLAB Function  Commented=through  TreatAsAtomicUnit=on
  MATLAB Function1 : MATLAB Function  Commented=through  TreatAsAtomicUnit=on
  Mux : Mux  Inputs=2
  Mux1 : Mux  Inputs=2
  Relational Operator : RelationalOperator  OutDataTypeStr=float('double')  InputSameDT=off
  Relational Operator1 : RelationalOperator  OutDataTypeStr=float('double')  InputSameDT=off
  Rounding Function1 : Rounding  Operator=round
  Rounding Function2 : Rounding  Operator=round
  Rtot_pu1 : Gain  Gain=Nb_PM  SaturateOnIntegerOverflow=on  OutDataTypeStr=Inherit: Same as input  ParamDataTypeStr=Inherit: Same as input
  Rtot_pu2 : Gain  Gain=Nb_PM  SaturateOnIntegerOverflow=on  OutDataTypeStr=Inherit: Same as input  ParamDataTypeStr=Inherit: Same as input
  Saturation : Saturate  UpperLimit=Nb_PM  LowerLimit=0
  Saturation1 : Saturate  UpperLimit=Nb_PM  LowerLimit=0
  Sum : Sum  Inputs=|-+
  Sum1 : Sum  Inputs=|-+
  Pp : Outport  VectorParamsAs1DForOutWhenUnconnected=off
  Pm : Outport  Port=2  VectorParamsAs1DForOutWhenUnconnected=off
  n_p : Outport  Port=3  VectorParamsAs1DForOutWhenUnconnected=off
  n_m : Outport  Port=4  VectorParamsAs1DForOutWhenUnconnected=off
  wires:
  Constant/1 -> Relational Operator/2
  Relational Operator/1 -> Logical Operator/1, Mux/1
  Logical Operator/1 -> Mux/2
  Mux/1 -> MATLAB Function/1(u)
  MATLAB Function/1(y) -> Pp/1
  Saturation1/1 -> n_p/1, Relational Operator/1
  Rtot_pu2/1 -> Sum/1
  Constant3/1 -> Sum/2
  Sum/1 -> Gain/1
  Gain/1 -> Rounding Function1/1
  Upref/1 -> Rtot_pu2/1
  Constant2/1 -> Relational Operator1/2
  Relational Operator1/1 -> Mux1/1, Logical Operator1/1
  Logical Operator1/1 -> Mux1/2
  Mux1/1 -> MATLAB Function1/1(u)
  MATLAB Function1/1(y) -> Pm/1
  Saturation/1 -> n_m/1, Relational Operator1/1
  Rounding Function1/1 -> Saturation1/1
  Rounding Function2/1 -> Saturation/1
  Sum1/1 -> Gain1/1
  Unref/1 -> Rtot_pu1/1
  Rtot_pu1/1 -> Sum1/1
  Constant1/1 -> Sum1/2
  Gain1/1 -> Rounding Function2/1

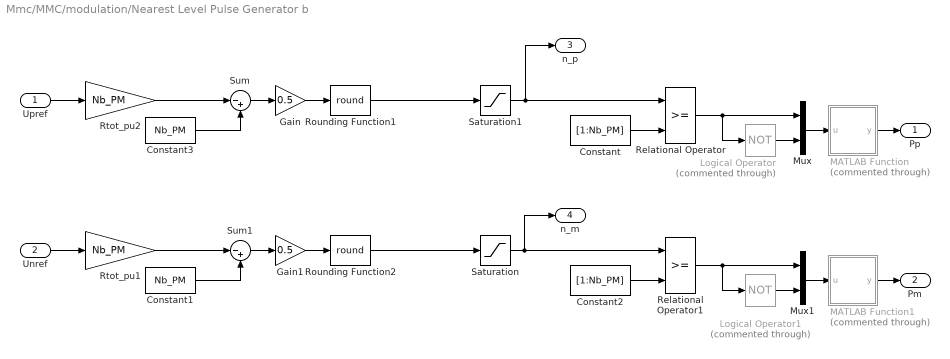
== system Mmc/MMC/modulation/Nearest Level Pulse Generator b ==
  Upref : Inport
  Unref : Inport  Port=2
  Constant : Constant  Value=[1:Nb_PM]
  Constant1 : Constant  Value=Nb_PM
  Constant2 : Constant  Value=[1:Nb_PM]
  Constant3 : Constant  Value=Nb_PM
  Gain : Gain  Gain=0.5
  Gain1 : Gain  Gain=0.5
  Logical Operator : Logic  Commented=through  Operator=NOT  AllPortsSameDT=off  OutDataTypeStr=float('double')
  Logical Operator1 : Logic  Commented=through  Operator=NOT  AllPortsSameDT=off  OutDataTypeStr=float('double')
  MATLAB Function : MATLAB Function  Commented=through  TreatAsAtomicUnit=on
  MATLAB Function1 : MATLAB Function  Commented=through  TreatAsAtomicUnit=on
  Mux : Mux  Inputs=2
  Mux1 : Mux  Inputs=2
  Relational Operator : RelationalOperator  OutDataTypeStr=float('double')  InputSameDT=off
  Relational Operator1 : RelationalOperator  OutDataTypeStr=float('double')  InputSameDT=off
  Rounding Function1 : Rounding  Operator=round
  Rounding Function2 : Rounding  Operator=round
  Rtot_pu1 : Gain  Gain=Nb_PM  SaturateOnIntegerOverflow=on  OutDataTypeStr=Inherit: Same as input  ParamDataTypeStr=Inherit: Same as input
  Rtot_pu2 : Gain  Gain=Nb_PM  SaturateOnIntegerOverflow=on  OutDataTypeStr=Inherit: Same as input  ParamDataTypeStr=Inherit: Same as input
  Saturation : Saturate  UpperLimit=Nb_PM  LowerLimit=0
  Saturation1 : Saturate  UpperLimit=Nb_PM  LowerLimit=0
  Sum : Sum  Inputs=|-+
  Sum1 : Sum  Inputs=|-+
  Pp : Outport  VectorParamsAs1DForOutWhenUnconnected=off
  Pm : Outport  Port=2  VectorParamsAs1DForOutWhenUnconnected=off
  n_p : Outport  Port=3  VectorParamsAs1DForOutWhenUnconnected=off
  n_m : Outport  Port=4  VectorParamsAs1DForOutWhenUnconnected=off
  wires:
  Gain1/1 -> Rounding Function2/1
  Constant1/1 -> Sum1/2
  Rtot_pu1/1 -> Sum1/1
  Unref/1 -> Rtot_pu1/1
  Sum1/1 -> Gain1/1
  Rounding Function2/1 -> Saturation/1
  Rounding Function1/1 -> Saturation1/1
  Saturation/1 -> Relational Operator1/1, n_m/1
  MATLAB Function1/1(y) -> Pm/1
  Mux1/1 -> MATLAB Function1/1(u)
  Logical Operator1/1 -> Mux1/2
  Relational Operator1/1 -> Logical Operator1/1, Mux1/1
  Constant2/1 -> Relational Operator1/2
  Upref/1 -> Rtot_pu2/1
  Gain/1 -> Rounding Function1/1
  Sum/1 -> Gain/1
  Constant3/1 -> Sum/2
  Rtot_pu2/1 -> Sum/1
  Saturation1/1 -> Relational Operator/1, n_p/1
  MATLAB Function/1(y) -> Pp/1
  Mux/1 -> MATLAB Function/1(u)
  Logical Operator/1 -> Mux/2
  Relational Operator/1 -> Mux/1, Logical Operator/1
  Constant/1 -> Relational Operator/2

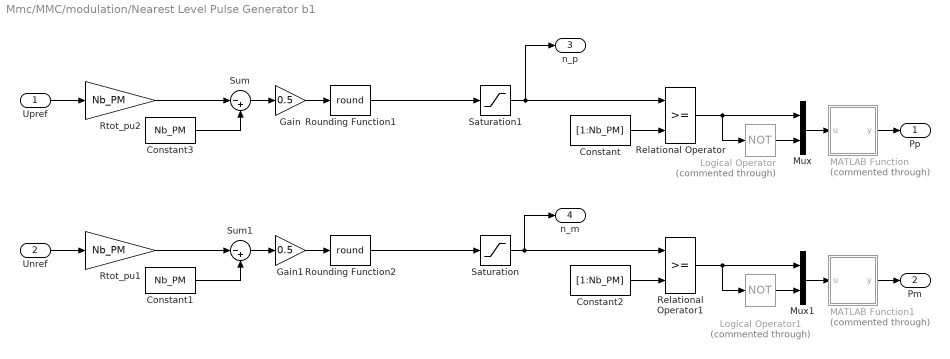
== system Mmc/MMC/modulation/Nearest Level Pulse Generator b1 ==
  Upref : Inport
  Unref : Inport  Port=2
  Constant : Constant  Value=[1:Nb_PM]
  Constant1 : Constant  Value=Nb_PM
  Constant2 : Constant  Value=[1:Nb_PM]
  Constant3 : Constant  Value=Nb_PM
  Gain : Gain  Gain=0.5
  Gain1 : Gain  Gain=0.5
  Logical Operator : Logic  Commented=through  Operator=NOT  AllPortsSameDT=off  OutDataTypeStr=float('double')
  Logical Operator1 : Logic  Commented=through  Operator=NOT  AllPortsSameDT=off  OutDataTypeStr=float('double')
  MATLAB Function : MATLAB Function  Commented=through  TreatAsAtomicUnit=on
  MATLAB Function1 : MATLAB Function  Commented=through  TreatAsAtomicUnit=on
  Mux : Mux  Inputs=2
  Mux1 : Mux  Inputs=2
  Relational Operator : RelationalOperator  OutDataTypeStr=float('double')  InputSameDT=off
  Relational Operator1 : RelationalOperator  OutDataTypeStr=float('double')  InputSameDT=off
  Rounding Function1 : Rounding  Operator=round
  Rounding Function2 : Rounding  Operator=round
  Rtot_pu1 : Gain  Gain=Nb_PM  SaturateOnIntegerOverflow=on  OutDataTypeStr=Inherit: Same as input  ParamDataTypeStr=Inherit: Same as input
  Rtot_pu2 : Gain  Gain=Nb_PM  SaturateOnIntegerOverflow=on  OutDataTypeStr=Inherit: Same as input  ParamDataTypeStr=Inherit: Same as input
  Saturation : Saturate  UpperLimit=Nb_PM  LowerLimit=0
  Saturation1 : Saturate  UpperLimit=Nb_PM  LowerLimit=0
  Sum : Sum  Inputs=|-+
  Sum1 : Sum  Inputs=|-+
  Pp : Outport  VectorParamsAs1DForOutWhenUnconnected=off
  Pm : Outport  Port=2  VectorParamsAs1DForOutWhenUnconnected=off
  n_p : Outport  Port=3  VectorParamsAs1DForOutWhenUnconnected=off
  n_m : Outport  Port=4  VectorParamsAs1DForOutWhenUnconnected=off
  wires:
  Gain1/1 -> Rounding Function2/1
  Constant1/1 -> Sum1/2
  Rtot_pu1/1 -> Sum1/1
  Unref/1 -> Rtot_pu1/1
  Sum1/1 -> Gain1/1
  Rounding Function2/1 -> Saturation/1
  Rounding Function1/1 -> Saturation1/1
  Saturation/1 -> Relational Operator1/1, n_m/1
  MATLAB Function1/1(y) -> Pm/1
  Mux1/1 -> MATLAB Function1/1(u)
  Logical Operator1/1 -> Mux1/2
  Relational Operator1/1 -> Logical Operator1/1, Mux1/1
  Constant2/1 -> Relational Operator1/2
  Upref/1 -> Rtot_pu2/1
  Gain/1 -> Rounding Function1/1
  Sum/1 -> Gain/1
  Constant3/1 -> Sum/2
  Rtot_pu2/1 -> Sum/1
  Saturation1/1 -> Relational Operator/1, n_p/1
  MATLAB Function/1(y) -> Pp/1
  Mux/1 -> MATLAB Function/1(u)
  Logical Operator/1 -> Mux/2
  Relational Operator/1 -> Mux/1, Logical Operator/1
  Constant/1 -> Relational Operator/2

== system Mmc/MMC/modulation/Sorting na ==
  note: A secrect, unintelligible, confusing and insrutable function with \if inside \for inside \if inside \if inside \if
  Usm : Inport
  N : Inport  Port=2
  Iarm : Inport  Port=3
  Constant : Constant  Value=SigmaM
  Logical Operator : Logic  Operator=NOT  AllPortsSameDT=off  OutDataTypeStr=float('double')
  MATLAB Function : MATLAB Function  TreatAsAtomicUnit=on
  MATLAB Function1 : MATLAB Function  TreatAsAtomicUnit=on
  Memory : Memory  InitialCondition=logical(zeros(Nb_PM, 1))  InheritSampleTime=on
  Mux : Mux  Inputs=2
  firing : Outport
  wires:
  MATLAB Function1/1(y) -> firing/1
  Logical Operator/1 -> Mux/2
  MATLAB Function/1(Ons_next) -> Mux/1, Logical Operator/1, Memory/1
  Mux/1 -> MATLAB Function1/1(u)
  Usm/1 -> MATLAB Function/1(Usm)
  Constant/1 -> MATLAB Function/3(Sigmam)
  N/1 -> MATLAB Function/2(N)
  Memory/1 -> MATLAB Function/5(Ons)
  Iarm/1 -> MATLAB Function/4(Iarm)

== system Mmc/MMC/modulation/Sorting nb ==
  note: A secrect, unintelligible, confusing and insrutable function with \if inside \for inside \if inside \if inside \if
  Usm : Inport
  N : Inport  Port=2
  Iarm : Inport  Port=3
  Constant : Constant  Value=SigmaM
  Logical Operator : Logic  Operator=NOT  AllPortsSameDT=off  OutDataTypeStr=float('double')
  MATLAB Function : MATLAB Function  TreatAsAtomicUnit=on
  MATLAB Function1 : MATLAB Function  TreatAsAtomicUnit=on
  Memory : Memory  InitialCondition=logical(zeros(Nb_PM, 1))  InheritSampleTime=on
  Mux : Mux  Inputs=2
  firing : Outport
  wires:
  MATLAB Function1/1(y) -> firing/1
  Logical Operator/1 -> Mux/2
  MATLAB Function/1(Ons_next) -> Mux/1, Logical Operator/1, Memory/1
  Mux/1 -> MATLAB Function1/1(u)
  Usm/1 -> MATLAB Function/1(Usm)
  Constant/1 -> MATLAB Function/3(Sigmam)
  N/1 -> MATLAB Function/2(N)
  Memory/1 -> MATLAB Function/5(Ons)
  Iarm/1 -> MATLAB Function/4(Iarm)

== system Mmc/MMC/modulation/Sorting nc ==
  note: A secrect, unintelligible, confusing and insrutable function with \if inside \for inside \if inside \if inside \if
  Usm : Inport
  N : Inport  Port=2
  Iarm : Inport  Port=3
  Constant : Constant  Value=SigmaM
  Logical Operator : Logic  Operator=NOT  AllPortsSameDT=off  OutDataTypeStr=float('double')
  MATLAB Function : MATLAB Function  TreatAsAtomicUnit=on
  MATLAB Function1 : MATLAB Function  TreatAsAtomicUnit=on
  Memory : Memory  InitialCondition=logical(zeros(Nb_PM, 1))  InheritSampleTime=on
  Mux : Mux  Inputs=2
  firing : Outport
  wires:
  MATLAB Function1/1(y) -> firing/1
  Logical Operator/1 -> Mux/2
  MATLAB Function/1(Ons_next) -> Mux/1, Logical Operator/1, Memory/1
  Mux/1 -> MATLAB Function1/1(u)
  Usm/1 -> MATLAB Function/1(Usm)
  Constant/1 -> MATLAB Function/3(Sigmam)
  N/1 -> MATLAB Function/2(N)
  Memory/1 -> MATLAB Function/5(Ons)
  Iarm/1 -> MATLAB Function/4(Iarm)

== system Mmc/MMC/modulation/Sorting pa ==
  note: A secrect, unintelligible, confusing and insrutable function with \if inside \for inside \if inside \if inside \if
  Usm : Inport
  N : Inport  Port=2
  Iarm : Inport  Port=3
  Constant : Constant  Value=SigmaM
  Logical Operator : Logic  Operator=NOT  AllPortsSameDT=off  OutDataTypeStr=float('double')
  MATLAB Function : MATLAB Function  TreatAsAtomicUnit=on
  MATLAB Function1 : MATLAB Function  TreatAsAtomicUnit=on
  Memory : Memory  InitialCondition=logical(zeros(Nb_PM, 1))  InheritSampleTime=on
  Mux : Mux  Inputs=2
  firing : Outport
  wires:
  Iarm/1 -> MATLAB Function/4(Iarm)
  Memory/1 -> MATLAB Function/5(Ons)
  N/1 -> MATLAB Function/2(N)
  Constant/1 -> MATLAB Function/3(Sigmam)
  Usm/1 -> MATLAB Function/1(Usm)
  Mux/1 -> MATLAB Function1/1(u)
  MATLAB Function/1(Ons_next) -> Memory/1, Logical Operator/1, Mux/1
  Logical Operator/1 -> Mux/2
  MATLAB Function1/1(y) -> firing/1

== system Mmc/MMC/modulation/Sorting pb ==
  note: A secrect, unintelligible, confusing and insrutable function with \if inside \for inside \if inside \if inside \if
  Usm : Inport
  N : Inport  Port=2
  Iarm : Inport  Port=3
  Constant : Constant  Value=SigmaM
  Logical Operator : Logic  Operator=NOT  AllPortsSameDT=off  OutDataTypeStr=float('double')
  MATLAB Function : MATLAB Function  TreatAsAtomicUnit=on
  MATLAB Function1 : MATLAB Function  TreatAsAtomicUnit=on
  Memory : Memory  InitialCondition=logical(zeros(Nb_PM, 1))  InheritSampleTime=on
  Mux : Mux  Inputs=2
  firing : Outport
  wires:
  Iarm/1 -> MATLAB Function/4(Iarm)
  Memory/1 -> MATLAB Function/5(Ons)
  N/1 -> MATLAB Function/2(N)
  Constant/1 -> MATLAB Function/3(Sigmam)
  Usm/1 -> MATLAB Function/1(Usm)
  Mux/1 -> MATLAB Function1/1(u)
  MATLAB Function/1(Ons_next) -> Memory/1, Logical Operator/1, Mux/1
  Logical Operator/1 -> Mux/2
  MATLAB Function1/1(y) -> firing/1

== system Mmc/MMC/modulation/Sorting pc ==
  note: A secrect, unintelligible, confusing and insrutable function with \if inside \for inside \if inside \if inside \if
  Usm : Inport
  N : Inport  Port=2
  Iarm : Inport  Port=3
  Constant : Constant  Value=SigmaM
  Logical Operator : Logic  Operator=NOT  AllPortsSameDT=off  OutDataTypeStr=float('double')
  MATLAB Function : MATLAB Function  TreatAsAtomicUnit=on
  MATLAB Function1 : MATLAB Function  TreatAsAtomicUnit=on
  Memory : Memory  InitialCondition=logical(zeros(Nb_PM, 1))  InheritSampleTime=on
  Mux : Mux  Inputs=2
  firing : Outport
  wires:
  Iarm/1 -> MATLAB Function/4(Iarm)
  Memory/1 -> MATLAB Function/5(Ons)
  N/1 -> MATLAB Function/2(N)
  Constant/1 -> MATLAB Function/3(Sigmam)
  Usm/1 -> MATLAB Function/1(Usm)
  Mux/1 -> MATLAB Function1/1(u)
  MATLAB Function/1(Ons_next) -> Memory/1, Logical Operator/1, Mux/1
  Logical Operator/1 -> Mux/2
  MATLAB Function1/1(y) -> firing/1

== system Mmc/MMC/modulation/Subsystem10 ==
  ref : Inport
  PWM Generator (Multilevel) : eePwmGeneratorMultilevel/PWM Generator (Multilevel)  topology=Full-bridge  Nsm=Nb_PM  Tper=1/fs  Ts=Ts_Power
  Scope : Scope
  Upper arm a : MATLAB Function  TreatAsAtomicUnit=on
  n_pwm : Outport
  wires:
  ref/1 -> PWM Generator (Multilevel)/1
  Upper arm a/1(n_pwm) -> n_pwm/1, Scope/1
  PWM Generator (Multilevel)/1 -> Upper arm a/1(signals)

== system Mmc/MMC/modulation/Subsystem11 ==
  ref : Inport
  PWM Generator (Multilevel) : eePwmGeneratorMultilevel/PWM Generator (Multilevel)  topology=Full-bridge  Nsm=Nb_PM  Tper=1/fs  Ts=Ts_Power
  Scope : Scope
  Upper arm a : MATLAB Function  TreatAsAtomicUnit=on
  n_pwm : Outport
  wires:
  PWM Generator (Multilevel)/1 -> Upper arm a/1(signals)
  Upper arm a/1(n_pwm) -> Scope/1, n_pwm/1
  ref/1 -> PWM Generator (Multilevel)/1

== system Mmc/MMC/modulation/Subsystem6 ==
  ref : Inport
  PWM Generator (Multilevel) : eePwmGeneratorMultilevel/PWM Generator (Multilevel)  topology=Full-bridge  Nsm=Nb_PM  Tper=1/fs  Ts=Ts_Power
  Scope : Scope
  Upper arm a : MATLAB Function  TreatAsAtomicUnit=on
  n_pwm : Outport
  wires:
  ref/1 -> PWM Generator (Multilevel)/1
  Upper arm a/1(n_pwm) -> n_pwm/1, Scope/1
  PWM Generator (Multilevel)/1 -> Upper arm a/1(signals)

== system Mmc/MMC/modulation/Subsystem7 ==
  ref : Inport
  PWM Generator (Multilevel) : eePwmGeneratorMultilevel/PWM Generator (Multilevel)  topology=Full-bridge  Nsm=Nb_PM  Tper=1/fs  Ts=Ts_Power
  Scope : Scope
  Upper arm a : MATLAB Function  TreatAsAtomicUnit=on
  n_pwm : Outport
  wires:
  PWM Generator (Multilevel)/1 -> Upper arm a/1(signals)
  Upper arm a/1(n_pwm) -> Scope/1, n_pwm/1
  ref/1 -> PWM Generator (Multilevel)/1

== system Mmc/MMC/modulation/Subsystem8 ==
  ref : Inport
  PWM Generator (Multilevel) : eePwmGeneratorMultilevel/PWM Generator (Multilevel)  topology=Full-bridge  Nsm=Nb_PM  Tper=1/fs  Ts=Ts_Power
  Scope : Scope
  Upper arm a : MATLAB Function  TreatAsAtomicUnit=on
  n_pwm : Outport
  wires:
  ref/1 -> PWM Generator (Multilevel)/1
  Upper arm a/1(n_pwm) -> n_pwm/1, Scope/1
  PWM Generator (Multilevel)/1 -> Upper arm a/1(signals)

== system Mmc/MMC/modulation/Subsystem9 ==
  ref : Inport
  PWM Generator (Multilevel) : eePwmGeneratorMultilevel/PWM Generator (Multilevel)  topology=Full-bridge  Nsm=Nb_PM  Tper=1/fs  Ts=Ts_Power
  Scope : Scope
  Upper arm a : MATLAB Function  TreatAsAtomicUnit=on
  n_pwm : Outport
  wires:
  PWM Generator (Multilevel)/1 -> Upper arm a/1(signals)
  Upper arm a/1(n_pwm) -> Scope/1, n_pwm/1
  ref/1 -> PWM Generator (Multilevel)/1

== matlab function Mmc/MMC/modulation/Subsystem9/Upper arm a ==
  data: signals input; n_pwm output
function n_pwm = PWM(signals)
% Name: PWM
% Input: the PWM gate signal of one arm.
%        40 signals with 0 or 1 
% Output: the number of activated submodels in one arm
%         0<Int(n_pwm)<20
% Discription: Get the number of activated submodels from the PWM gate
% signals

    % Identify if there is 40 signal inputs
    if length(signals) ~= 8
        error('Input must be a vector with exactly 40 elements.');
    end
    % Select the odd signal (the gate signal for upper side switch)
    %Sig_up = signals(1:2:end);
    counter = 0;
    if signals(1)==1 && signals(3)==1
        counter = counter + 1;
    end
    if signals(2)==1 && signals(4)==1
        counter = counter + 1;
    end
    if signals(5)==1 && signals(7)==1
        counter = counter + 1;
    end
    if signals(6)==1 && signals(8)==1
        counter = counter + 1;
    end

    % Count how many submodel is activated
    n_pwm = 2 - counter;%2 - sum(Sig_up);
    %counter = 0;
end

== matlab function Mmc/MMC/modulation/Nearest Level Pulse Generator a /MATLAB Function1 ==
  data: u input; y output
function y = FiringSorting(u)
    y = u;
    for i = 1: length(u)
        if mod(i, 2) == 1
            y(i) = u(int16(i/2));
        else
            y(i) = u(int16(i/2+length(u)/2));
        end
    end
end

== matlab function Mmc/MMC/modulation/Sorting na/MATLAB Function ==
  data: Usm input; N input; Ons_next output; Sigmam input; Iarm input; Ons input
function Ons_next = SmFiringSorting(Usm, N, Sigmam, Iarm, Ons)
    %%%
    % SmFiringSorting -- SM firing sorting. -- C.SI on 5th, Oct.
    %% Inputs:
    % Usm - capacitor voltage on each SM;
    % N - number of SMs that needed to fire up;
    % Sigmam [%] - Maximum allowed voltage unbalance rate;
    % Iarm - arm current;
    % Ons (boolean) - indicate those SM(s) who are in series with the
    % source in the last control period;
    %% Outputs:
    % Ons_now (boolean) - indicate those SM(s) who should be in series with 
    % the source in this control period;
    %%%
    
    % number of SMs
    Nb = length(Usm);
    % initialize the on-state boolean array
    Ons_next = zeros(Nb, 1); 
    % rank the SMs in the order of descendance
    [~, order] = sort(Usm, 'descend');
    
    if max(abs(1-Usm)) > Sigmam/100
        % Over the maximum unbalance acceptance
        if Iarm > 0
            % charge the capacitors with lowest voltages
            Ons_next(order(Nb-N+1: Nb)) = ~Ons_next(order(Nb-N+1: Nb));
        else
            % discharge the capacitors with highest voltages
            Ons_next(order(1: N)) = ~Ons_next(order(1: N));
        end

    else
        if N-sum(Ons) ==  0
            % if we don't need to change the number of SM that is on
            Ons_next = Ons;
        
        elseif N-sum(Ons) > 0
            % if we need more SMs are to be on-state

            % number of SMs that needed to be changed the state
            DeltaN = N-sum(Ons);
            % keep previously being on SMs still being on
            Ons_next = Ons;

            if Iarm > 0
                % charge the capacitors with lowest voltages
                for i = 1: Nb
                    if DeltaN <= 0
                        break;
                    end
                    % if the SM is off and still need more SM
                    if Ons(order(Nb-i+1)) == false
                        DeltaN = DeltaN - 1;
                        Ons_next(order(Nb-i+1)) = true;
                    end
                end

            else
                % discharge the capacitors with highest voltages
                for i = 1: Nb
                    if DeltaN <= 0
                        break;
                    end
                    % if the SM is off and still need more SM
                    if Ons(order(i)) == false
                        DeltaN = DeltaN - 1;
                        Ons_next(order(i)) = true;
                    end
                end
            end

        else
            % if we need less SMs are to be on-state

            % number of SMs that needed to be changed the state
            DeltaN = sum(Ons)-N;
            % keep previously being on SMs still being on
            Ons_next = Ons;

            if Iarm > 0
                % remove the capacitor with highest voltage
                for i = 1: Nb
                    if DeltaN <= 0
                        break;
                    end
                    % if the SM is on and still need less SM
                    if Ons(order(i)) == true
                        DeltaN = DeltaN - 1;
                        Ons_next(order(i)) = false;
                    end
                end

            else
                % remove the capacitor with lowest voltage
                for i = 1: Nb
                    if DeltaN <= 0
                        break;
                    end
                    % if the SM is on and still need less SM
                    if Ons(order(Nb-i+1)) == true
                        DeltaN = DeltaN - 1;
                        Ons_next(order(Nb-i+1)) = false;
                    end
                end
            end
        end
    end
end

== matlab function Mmc/MMC/modulation/Sorting na/MATLAB Function1 ==
  data: u input; y output
function y = FiringSorting(u)
    y = u;
    for i = 1: length(u)
        if mod(i, 2) == 1
            y(i) = u(int16(i/2));
        else
            y(i) = u(int16(i/2+length(u)/2));
        end
    end
end
